simulink model "model_6dof"  (R2025b)
settings: Solver=ode45  StartTime=0.0  StopTime=T_sim  RelTol=1e-6
undefined symbols (not defined in the file or in its folder): body_secondary, boresight_b, dist_amp, dist_amp_pos, dist_freq, dist_freq_pos, eta_att, eta_pos, hcw_accel_sl, IJ, J, K_att, K_pos, M_sat, omega_orb, phi_att, phi_pos, pointing_ref_gen_sl, q0, smc_attitude_sl, smc_translational_sl, u_sat, up_hint, w0, z0, z_r
libraries: vrlib x1
settings Model: Creator=franc  LastModifiedBy=franc

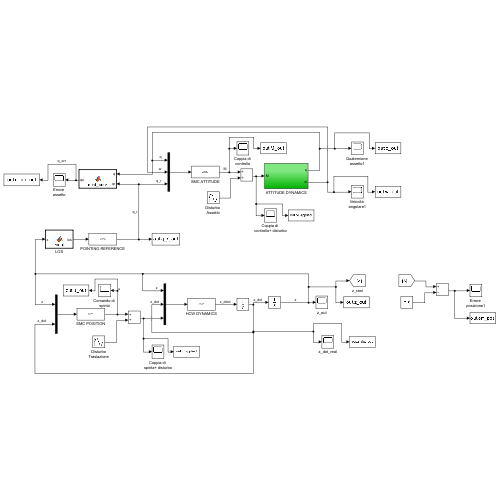
[thumbnail: Simulink's stored preview of the top-level diagram]
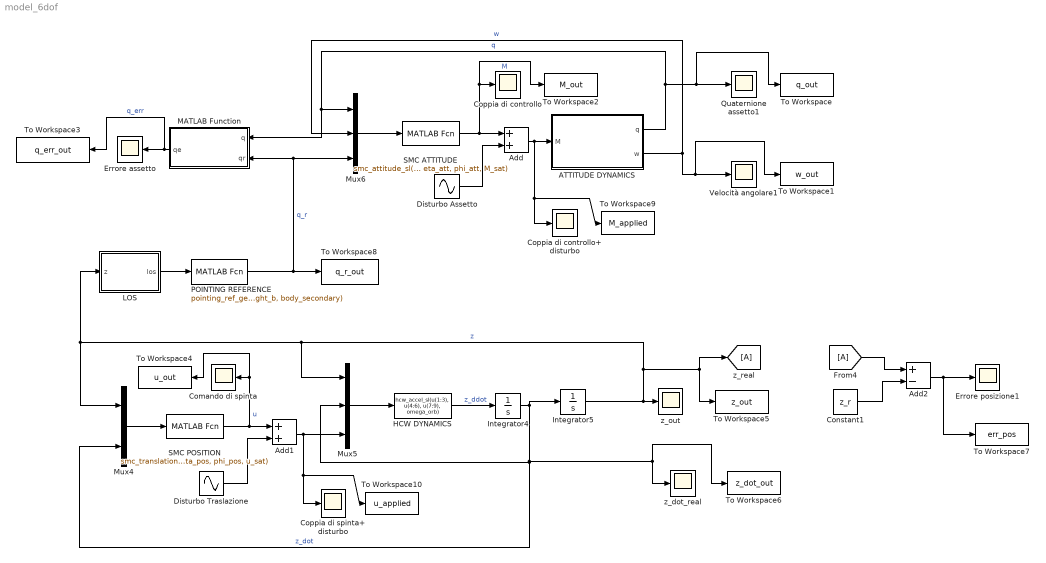
== system model_6dof ==
  ATTITUDE DYNAMICS : Subsystem
  Add : Sum
  Add1 : Sum
  Add2 : Sum  Inputs=+-
  Comando di spinta : Scope
      settings: ActiveDisplayYMinimum=-0.12069026490196488  ActiveDisplayYMaximum=0.11637453315057719  DataLoggingVariableName=ScopeData12
  Constant1 : Constant  Value=z_r
  Coppia di controllo : Scope
      settings: ActiveDisplayYMinimum=-0.10652475572965329  ActiveDisplayYMaximum=0.644368793227296  DataLoggingVariableName=ScopeData13
  Coppia di controllo+ disturbo : Scope
      settings: ActiveDisplayYMinimum=-0.10652475572965329  ActiveDisplayYMaximum=0.644368793227296
  Coppia di spinta+ disturbo : Scope
      settings: ActiveDisplayYMinimum=-0.10652475572965329  ActiveDisplayYMaximum=0.644368793227296
  Disturbo Traslazione : Sin  Amplitude=dist_amp_pos*[1;0.6;0.3]  Frequency=dist_freq_pos  SampleTime=0
  Disturbo Assetto : Sin  Amplitude=dist_amp*[1;0.6;0.3]  Frequency=dist_freq  SampleTime=0
  Errore assetto : Scope
      settings: ActiveDisplayYMinimum=-0.92961725275602469  ActiveDisplayYMaximum=1.2144019154276502  DataLoggingVariableName=ScopeData14
  Errore posizione1 : Scope
      settings: DataLoggingVariableName=ScopeData15
  From4 : From
  HCW DYNAMICS : MATLABFcn  MATLABFcn=hcw_accel_sl(u(1:3), u(4:6), u(7:9), omega_orb)
  Integrator4 : Integrator  InitialCondition=w0
  Integrator5 : Integrator  InitialCondition=z0
  LOS : MATLAB Function  TreatAsAtomicUnit=on
  MATLAB Function : MATLAB Function  TreatAsAtomicUnit=on
  Mux4 : Mux  Inputs=2
  Mux5 : Mux  Inputs=3
  Mux6 : Mux  Inputs=3
  POINTING REFERENCE : MATLABFcn  MATLABFcn=pointing_ref_gen_sl(u, up_hint, boresight_b, body_secondary)
  Quaternione assetto1 : Scope
      settings: ActiveDisplayYMinimum=-0.12609336200782117  ActiveDisplayYMaximum=1.1251214846675357  DataLoggingVariableName=ScopeData16
  SMC ATTITUDE : MATLABFcn  MATLABFcn=smc_attitude_sl(u(1:4), u(5:7), u(8:11), [0;0;0], J, K_att, eta_att, phi_att, M_sat)
  SMC POSITION : MATLABFcn  MATLABFcn=smc_translational_sl(u(1:3), u(4:6), z_r, omega_orb, K_pos, eta_pos, phi_pos, u_sat)
  To Workspace : ToWorkspace  VariableName=q_out  SaveFormat=Timeseries  SampleTime=-1
  To Workspace1 : ToWorkspace  VariableName=w_out  SaveFormat=Timeseries  SampleTime=-1
  To Workspace10 : ToWorkspace  VariableName=u_applied  SaveFormat=Timeseries  SampleTime=-1
  To Workspace2 : ToWorkspace  VariableName=M_out  SaveFormat=Timeseries  SampleTime=-1
  To Workspace3 : ToWorkspace  VariableName=q_err_out  SaveFormat=Timeseries  SampleTime=-1
  To Workspace4 : ToWorkspace  VariableName=u_out  SaveFormat=Timeseries  SampleTime=-1
  To Workspace5 : ToWorkspace  VariableName=z_out  SaveFormat=Timeseries  SampleTime=-1
  To Workspace6 : ToWorkspace  VariableName=z_dot_out  SaveFormat=Timeseries  SampleTime=-1
  To Workspace7 : ToWorkspace  VariableName=err_pos  SaveFormat=Timeseries  SampleTime=-1
  To Workspace8 : ToWorkspace  VariableName=q_r_out  SaveFormat=Timeseries  SampleTime=-1
  To Workspace9 : ToWorkspace  VariableName=M_applied  SaveFormat=Timeseries  SampleTime=-1
  Velocità angolare1 : Scope
      settings: ActiveDisplayYMinimum=-0.0021434976653219194  ActiveDisplayYMaximum=0.018684289861101981  DataLoggingVariableName=ScopeData19
  z_dot_real : Scope
      settings: DataLoggingVariableName=ScopeData18
  z_out : Scope
      settings: ActiveDisplayYMinimum=-58.749999999999915  ActiveDisplayYMaximum=28.749999999999218  DataLoggingVariableName=ScopeData17
  z_real : Goto
  wires:
  SMC POSITION/1 -> Add1/1, To Workspace4/1, Comando di spinta/1  "u"
  Add2/1 -> To Workspace7/1, Errore posizione1/1
  Mux4/1 -> SMC POSITION/1
  LOS/1(los) -> POINTING REFERENCE/1
  Integrator4/1 -> Integrator5/1, Mux4/2, Mux5/2, z_dot_real/1, To Workspace6/1  "z_dot"
  Integrator5/1 -> Mux5/1, LOS/1(z), Mux4/1, To Workspace5/1, z_real/1, z_out/1  "z"
  Mux6/1 -> SMC ATTITUDE/1
  SMC ATTITUDE/1 -> Add/1, To Workspace2/1, Coppia di controllo/1  "M"
  ATTITUDE DYNAMICS/1(q) -> MATLAB Function/1(q), Mux6/1, To Workspace/1, Quaternione assetto1/1  "q"
  MATLAB Function/1(qe) -> To Workspace3/1, Errore assetto/1  "q_err"
  POINTING REFERENCE/1 -> Mux6/3, MATLAB Function/2(qr), To Workspace8/1  "q_r"
  Mux5/1 -> HCW DYNAMICS/1
  HCW DYNAMICS/1 -> Integrator4/1  "z_ddot"
  ATTITUDE DYNAMICS/2(w) -> To Workspace1/1, Velocità angolare1/1, Mux6/2  "w"
  From4/1 -> Add2/1
  Constant1/1 -> Add2/2
  Disturbo Assetto/1 -> Add/2
  Add/1 -> To Workspace9/1, Coppia di controllo+ disturbo/1, ATTITUDE DYNAMICS/1(M)
  Add1/1 -> To Workspace10/1, Coppia di spinta+ disturbo/1, Mux5/3
  Disturbo Traslazione/1 -> Add1/2

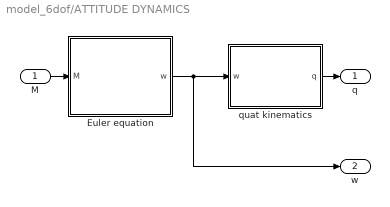
== system model_6dof/ATTITUDE DYNAMICS ==
  M : Inport
  Euler equation : Subsystem
  quat kinematics : Subsystem  AncestorBlock=lib_rotations_2014/quat kinematics
  q : Outport
  w : Outport  Port=2
  wires:
  M/1 -> Euler equation/1(M)
  Euler equation/1(w) -> w/1, quat kinematics/1(w)
  quat kinematics/1(q) -> q/1

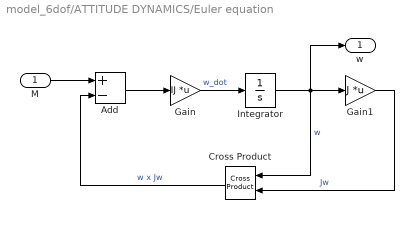
== system model_6dof/ATTITUDE DYNAMICS/Euler equation ==
  M : Inport
  Add : Sum  Inputs=+-
  Cross Product : vrlib/Utilities/Cross Product
  Gain : Gain  Gain=IJ  Multiplication=Matrix(K*u)
  Gain1 : Gain  Gain=J  Multiplication=Matrix(K*u)
  Integrator : Integrator  InitialCondition=w0
  w : Outport  VectorParamsAs1DForOutWhenUnconnected=off
  wires:
  M/1 -> Add/1
  Integrator/1 -> Gain1/1, w/1, Cross Product/1  "w"
  Gain/1 -> Integrator/1  "w_dot"
  Gain1/1 -> Cross Product/2  "Jw"
  Add/1 -> Gain/1
  Cross Product/1 -> Add/2  "w x Jw"

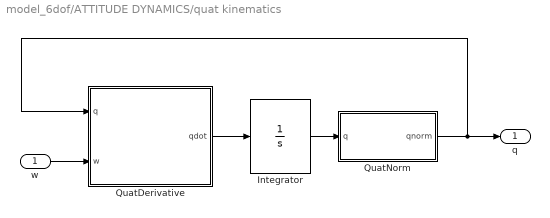
== system model_6dof/ATTITUDE DYNAMICS/quat kinematics ==
  w : Inport  PortDimensions=3
  Integrator : Integrator  InitialCondition=q0
  QuatDerivative : MATLAB Function  TreatAsAtomicUnit=on
  QuatNorm : MATLAB Function  TreatAsAtomicUnit=on
  q : Outport  PortDimensions=4  VectorParamsAs1DForOutWhenUnconnected=off
  wires:
  w/1 -> QuatDerivative/2(w)
  QuatDerivative/1(qdot) -> Integrator/1
  QuatNorm/1(qnorm) -> QuatDerivative/1(q), q/1
  Integrator/1 -> QuatNorm/1(q)

== matlab function model_6dof/ATTITUDE DYNAMICS/quat kinematics/QuatDerivative ==
  data: q input; qdot output; w input
function qdot = QuatDerivative(q,w)
    omegaq = [0; w];
    Q = [q(1) -q(2) -q(3) -q(4);
         q(2) q(1) -q(4) q(3);
         q(3) q(4) q(1) -q(2);
         q(4) -q(3) q(2) q(1)];
    qdot = Q*omegaq/2;
end

== matlab function model_6dof/ATTITUDE DYNAMICS/quat kinematics/QuatNorm ==
  data: q input; qnorm output
function qnorm = QuatNorm(q)
    qnorm = zeros(4,1);
    q2 = sqrt(q'*q);
    qnorm = q/q2;
end

== matlab function model_6dof/LOS ==
  data: z input; los output
function los = los_sl(z)

    r = -z;
    n = norm(r);
    
    if n > 1e-9
        los = r/n;
    else
        los = [1;0;0];
    end

end

== matlab function model_6dof/MATLAB Function ==
  data: q input; qr input; qe output
function qe  = quat_error(q, qr)
% QUAT_ERROR Compute attitude error between two unit quaternions
%
% Inputs:
%   qr = reference quaternion [4x1], scalar first
%   q  = current quaternion   [4x1], scalar first
%
% Outputs:
%   qe     = error quaternion
%   qe_vec = vector part of error quaternion

    % Normalize quaternions
    qr = qr / norm(qr);
    q  = q  / norm(q);

    % Ensure shortest rotation
    if dot(qr, q) < 0
        q = -q;
    end

    % Reference quaternion inverse
    qr_inv = [qr(1); -qr(2:4)];

    % Quaternion error
    qe = quatprod(qr_inv, q);
end


function r = quatprod(q, p)
% Quaternion product r = q ⊗ p
% Scalar-first convention

    q0 = q(1);
    qv = q(2:4);

    p0 = p(1);
    pv = p(2:4);

    r = [q0*p0 - dot(qv,pv);
         q0*pv + p0*qv + cross(qv,pv)];

end
